simulink model "ControlBrazo"  (R2025b)
settings: Solver=VariableStepAuto  StartTime=0.0  StopTime=50  RelTol=1e-3
values from neighbouring files (symbols this model uses):
  g = 9.81    [Datos (1).m]
  J = 0.006    [Datos (1).m]
  l = 0.3    [Datos (1).m]
  m = 1    [Datos (1).m]
libraries: fuzblock x1
settings Model: Creator=user

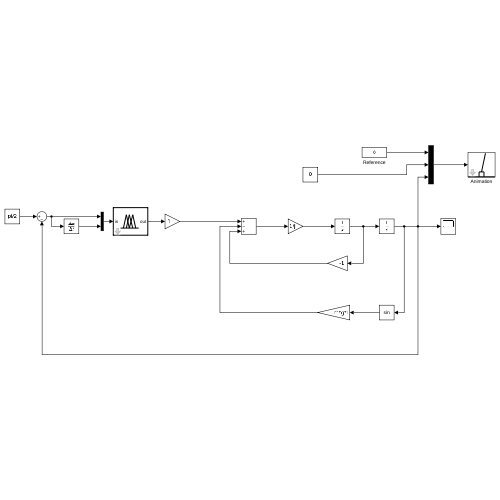
[thumbnail: Simulink's stored preview of the top-level diagram]
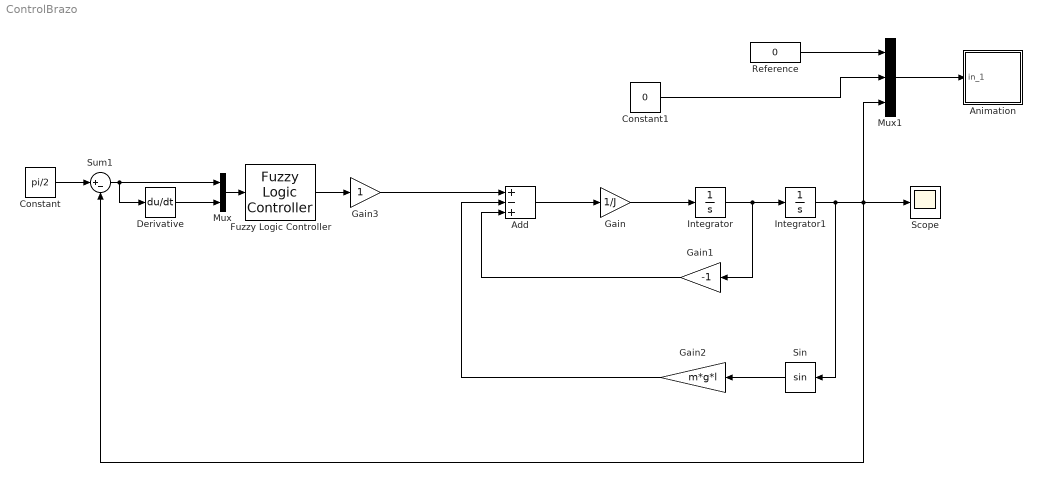
== system ControlBrazo ==
  Add : Sum  Inputs=+-+
  Animation : Subsystem  mask(Pendulum plot){RefBlock=Reference}
      mask prompts: RefBlock "DC reference signal block name:"
      mask help: Pendulum plot
      mask Help: Pendulum animation function using Handle graphics.
      mask Display: plot([-10 10],[0 0],[-2 -2 2 2],[0 1 1 0],[0 3],[1 5])
  Constant : Constant  Value=pi/2
  Constant1 : Constant  Value=0
  Derivative : Derivative
  Fuzzy Logic Controller : fuzblock/Fuzzy Logic  Controller  FIS='LogicaBrazo.fis'  OutputSampleNumber=101  DataType=double  UseLookupTable=off  NumBreakpoints=10  FuzzifiedInputs=off  RuleFiringStrengths=off  RuleOutputs=off  AggregatedOutputs=off  SimulateUsing=Interpreted execution  OutOfRangeInputValueMessage=warning  NoRuleFiredMessage=warning  EmptyOutputFuzzySetMessage=warning
  Gain : Gain  Gain=1/J
  Gain1 : Gain  Gain=-1
  Gain2 : Gain  Gain=m*g*l
  Gain3 : Gain
  Integrator : Integrator
  Integrator1 : Integrator  InitialCondition=2
  Mux : Mux  Inputs=2
  Mux1 : Mux  Inputs=3
  Reference : Constant  Value=0
  Scope : Scope
      settings: ActiveDisplayYMinimum=0.21187866318788506  ActiveDisplayYMaximum=2.3305798090737873
  Sin : Trigonometry
  Sum1 : Sum  Inputs=|+-
  wires:
  Add/1 -> Gain/1
  Gain/1 -> Integrator/1
  Integrator/1 -> Gain1/1, Integrator1/1
  Gain1/1 -> Add/3
  Gain2/1 -> Add/2
  Sin/1 -> Gain2/1
  Constant/1 -> Sum1/1
  Derivative/1 -> Mux/2
  Sum1/1 -> Derivative/1, Mux/1
  Mux/1 -> Fuzzy Logic Controller/1
  Gain3/1 -> Add/1
  Fuzzy Logic Controller/1 -> Gain3/1
  Integrator1/1 -> Sin/1, Mux1/3, Scope/1, Sum1/2
  Reference/1 -> Mux1/1
  Constant1/1 -> Mux1/2
  Mux1/1 -> Animation/1(in_1)

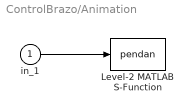
== system ControlBrazo/Animation ==
  in_1 : Inport
  Level-2 MATLAB S-Function : M-S-Function  FunctionName=pendan  Parameters=RefBlock
  wires:
  in_1/1 -> Level-2 MATLAB S-Function/1
